simulink model "sistema_fisico"  (R2023a)
settings: Solver=VariableStepAuto  StartTime=0.0  StopTime=10.0  RelTol=1e-3
undefined symbols (not defined in the file): b_hb, b_hEb, b_t, b_tb, b_tw, b_wu, bh_eq, bt_eq, i_h, i_t, Jh_eq, Jt_eq, k_tw, k_wu, m_t, r_hd, r_td
settings Model: Creator=renzo  LastModifiedBy=renzo

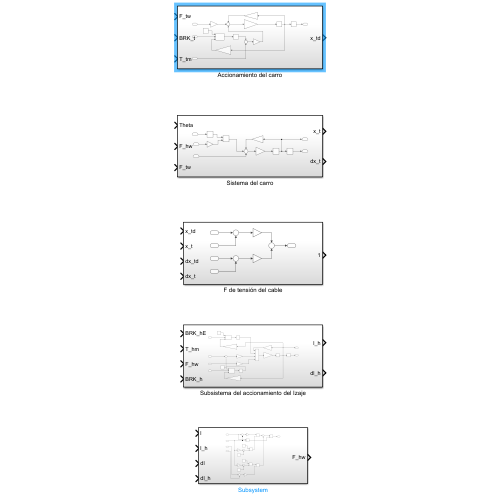
[thumbnail: Simulink's stored preview of the top-level diagram]
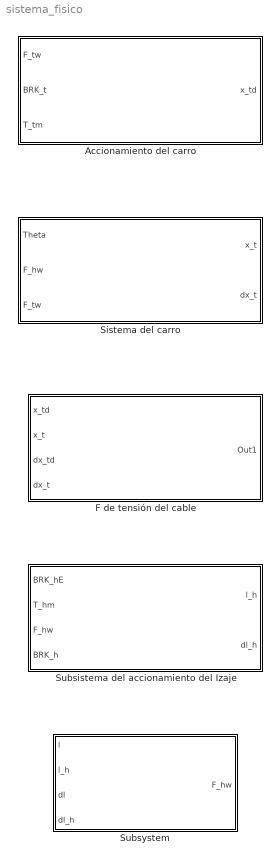
== system sistema_fisico ==
  Accionamiento del carro : Subsystem
  F de tensión del cable : Subsystem
  Sistema del carro : Subsystem
  Subsistema del accionamiento del Izaje : Subsystem
  Subsystem : Subsystem

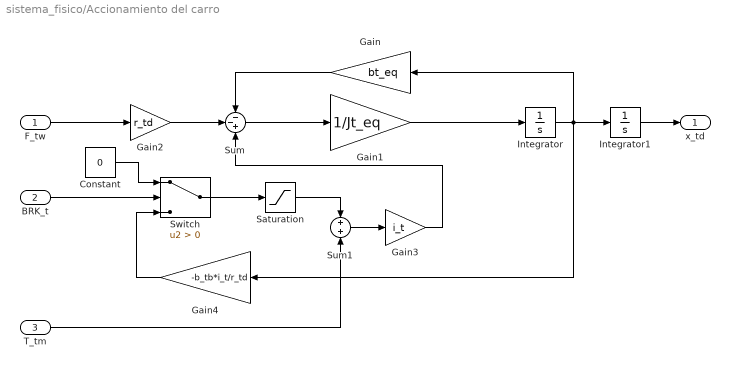
== system sistema_fisico/Accionamiento del carro ==
  F_tw : Inport
  BRK_t : Inport  Port=2
  T_tm : Inport  Port=3
  Constant : Constant  Value=0
  Gain : Gain  Gain=bt_eq
  Gain1 : Gain  Gain=1/Jt_eq
  Gain2 : Gain  Gain=r_td
  Gain3 : Gain  Gain=i_t
  Gain4 : Gain  Gain=-b_tb*i_t/r_td
  Integrator : Integrator
  Integrator1 : Integrator
  Saturation : Saturate
  Sum : Sum  Inputs=--+
  Sum1 : Sum
  Switch : Switch  Criteria=u2 > Threshold  SaturateOnIntegerOverflow=off  InputSameDT=off
  x_td : Outport
  wires:
  F_tw/1 -> Gain2/1
  Gain2/1 -> Sum/2
  Sum/1 -> Gain1/1
  Gain1/1 -> Integrator/1
  Integrator/1 -> Integrator1/1, Gain4/1, Gain/1
  Integrator1/1 -> x_td/1
  Gain/1 -> Sum/1
  Constant/1 -> Switch/1
  BRK_t/1 -> Switch/2
  Switch/1 -> Saturation/1
  Saturation/1 -> Sum1/1
  T_tm/1 -> Sum1/2
  Gain3/1 -> Sum/3
  Sum1/1 -> Gain3/1
  Gain4/1 -> Switch/3

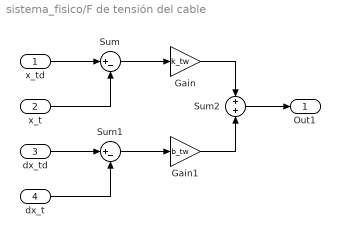
== system sistema_fisico/F de tensión del cable ==
  x_td : Inport
  x_t : Inport  Port=2
  dx_td : Inport  Port=3
  dx_t : Inport  Port=4
  Gain : Gain  Gain=k_tw
  Gain1 : Gain  Gain=b_tw
  Sum : Sum  Inputs=|+-
  Sum1 : Sum  Inputs=|+-
  Sum2 : Sum
  Out1 : Outport
  wires:
  x_td/1 -> Sum/1
  dx_td/1 -> Sum1/1
  x_t/1 -> Sum/2
  dx_t/1 -> Sum1/2
  Sum/1 -> Gain/1
  Sum1/1 -> Gain1/1
  Gain/1 -> Sum2/1
  Gain1/1 -> Sum2/2
  Sum2/1 -> Out1/1

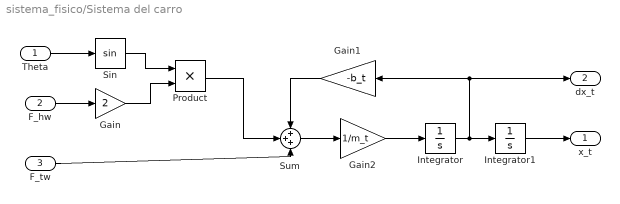
== system sistema_fisico/Sistema del carro ==
  Theta : Inport
  F_hw : Inport  Port=2
  F_tw : Inport  Port=3
  Gain : Gain  Gain=2
  Gain1 : Gain  Gain=-b_t
  Gain2 : Gain  Gain=1/m_t
  Integrator : Integrator
  Integrator1 : Integrator
  Product : Product
  Sin : Trigonometry
  Sum : Sum  Inputs=+++
  x_t : Outport
  dx_t : Outport  Port=2
  wires:
  Theta/1 -> Sin/1
  Sin/1 -> Product/1
  F_hw/1 -> Gain/1
  Gain/1 -> Product/2
  Product/1 -> Sum/2
  F_tw/1 -> Sum/3
  Gain1/1 -> Sum/1
  Sum/1 -> Gain2/1
  Gain2/1 -> Integrator/1
  Integrator/1 -> dx_t/1, Gain1/1, Integrator1/1
  Integrator1/1 -> x_t/1

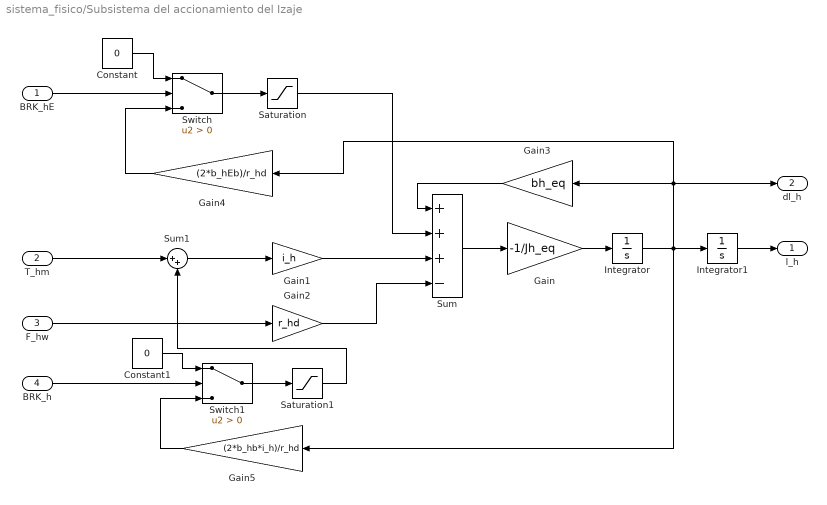
== system sistema_fisico/Subsistema del accionamiento del Izaje ==
  BRK_hE : Inport
  T_hm : Inport  Port=2
  F_hw : Inport  Port=3
  BRK_h : Inport  Port=4
  Constant : Constant  Value=0
  Constant1 : Constant  Value=0
  Gain : Gain  Gain=-1/Jh_eq
  Gain1 : Gain  Gain=i_h
  Gain2 : Gain  Gain=r_hd
  Gain3 : Gain  Gain=bh_eq
  Gain4 : Gain  Gain=(2*b_hEb)/r_hd
  Gain5 : Gain  Gain=(2*b_hb*i_h)/r_hd
  Integrator : Integrator
  Integrator1 : Integrator
  Saturation : Saturate
  Saturation1 : Saturate
  Sum : Sum  Inputs=+++-
  Sum1 : Sum  Inputs=|++
  Switch : Switch  Criteria=u2 > Threshold  SaturateOnIntegerOverflow=off  InputSameDT=off
  Switch1 : Switch  Criteria=u2 > Threshold  SaturateOnIntegerOverflow=off  InputSameDT=off
  l_h : Outport
  dl_h : Outport  Port=2
  wires:
  BRK_hE/1 -> Switch/2
  Constant/1 -> Switch/1
  Switch/1 -> Saturation/1
  Saturation/1 -> Sum/2
  T_hm/1 -> Sum1/1
  Gain1/1 -> Sum/3
  Sum1/1 -> Gain1/1
  Gain2/1 -> Sum/4
  F_hw/1 -> Gain2/1
  BRK_h/1 -> Switch1/2
  Constant1/1 -> Switch1/1
  Switch1/1 -> Saturation1/1
  Sum/1 -> Gain/1
  Gain3/1 -> Sum/1
  Gain/1 -> Integrator/1
  Integrator/1 -> dl_h/1, Gain4/1, Gain3/1, Integrator1/1, Gain5/1
  Integrator1/1 -> l_h/1
  Gain4/1 -> Switch/3
  Gain5/1 -> Switch1/3
  Saturation1/1 -> Sum1/2

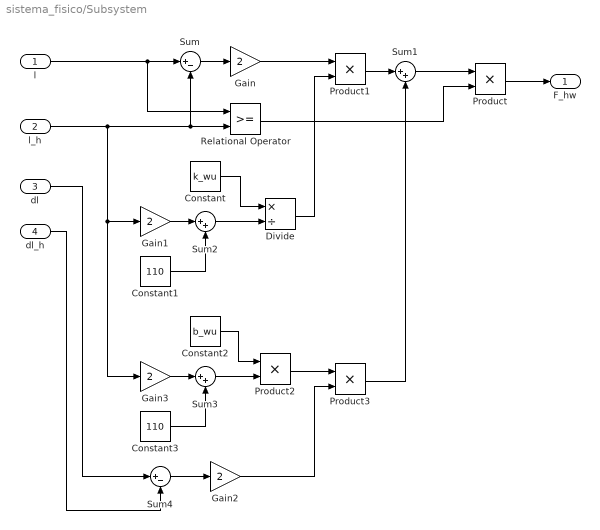
== system sistema_fisico/Subsystem ==
  l : Inport
  l_h : Inport  Port=2
  dl : Inport  Port=3
  dl_h : Inport  Port=4
  Constant : Constant  Value=k_wu
  Constant1 : Constant  Value=110
  Constant2 : Constant  Value=b_wu
  Constant3 : Constant  Value=110
  Divide : Product  Inputs=*/
  Gain{,1..3} (4 alike) : Gain  Gain=2
  Product{,1..3} (4 alike) : Product
  Relational Operator : RelationalOperator  OutDataTypeStr=boolean  RndMeth=Simplest  InputSameDT=off
  Sum : Sum  Inputs=|+-
  Sum1 : Sum  Inputs=|++
  Sum2 : Sum  Inputs=|++
  Sum3 : Sum  Inputs=|++
  Sum4 : Sum  Inputs=|+-
  F_hw : Outport
  wires:
  l/1 -> Relational Operator/1, Sum/1
  Sum/1 -> Gain/1
  Gain/1 -> Product1/1
  Product1/1 -> Sum1/1
  Product/1 -> F_hw/1
  Constant/1 -> Divide/1
  Gain1/1 -> Sum2/1
  Constant1/1 -> Sum2/2
  Sum2/1 -> Divide/2
  Divide/1 -> Product1/2
  Gain3/1 -> Sum3/1
  Constant3/1 -> Sum3/2
  Constant2/1 -> Product2/1
  l_h/1 -> Gain1/1, Gain3/1, Relational Operator/2, Sum/2
  Sum3/1 -> Product2/2
  Product2/1 -> Product3/1
  dl/1 -> Sum4/1
  dl_h/1 -> Sum4/2
  Sum4/1 -> Gain2/1
  Gain2/1 -> Product3/2
  Product3/1 -> Sum1/2
  Relational Operator/1 -> Product/2
  Sum1/1 -> Product/1
